simulink model "Sl_H_Infinity_Regulater"  (R2015a)
settings: Solver=FixedStepDiscrete  StartTime=0.0  StopTime=10.0  FixedStep=1  RelTol=1e-3
values from neighbouring files (symbols this model uses):
  kd = c2d(K,0.1)    [Sc_H_Infinity.m]
settings Model: CovSFcnEnable=off  Creator=jordan  LastModifiedBy=Vladislav
settings DataIOCC: SignalLoggingSaveFormat=ModelDataLogs
settings OptimizationCC: ExpressionDepthLimit=2147483647  OptimizeModelRefInitCode=on  LifeSpan=1
settings DebuggingCC: UnderspecifiedInitializationDetection=Classic  MergeDetectMultiDrivingBlocksExec=none  SolverPrmCheckMsg=warning  FcnCallInpInsideContextMsg=UseLocalSettings  StateNameClashWarn=warning
settings RTWCC: SystemTargetFile=ert.tlc  TemplateMakefile=ert_default_tmf  Description=Embedded Coder
settings CodeAppCC: IgnoreCustomStorageClasses=off
settings ERTTargetCC: ParMdlRefBuildCompliant=on  CompOptLevelCompliant=on  ConcurrentExecutionCompliant=on  ERTFirstTimeCompliant=on  SupportContinuousTime=off  SupportVariableSizeSignals=off  ModelStepFunctionPrototypeControlCompliant=on  CPPClassGenCompliant=on  InlinedParameterPlacement=Hierarchical  ERTCustomFileTemplate=example_file_process.tlc

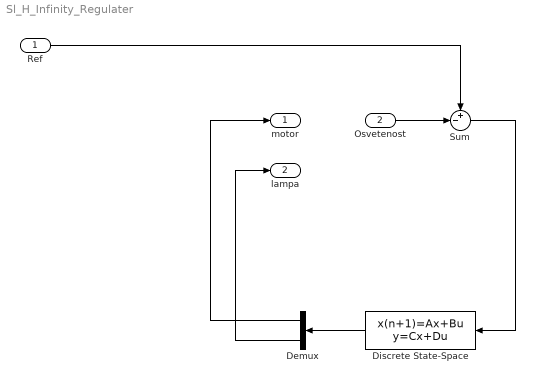
== system Sl_H_Infinity_Regulater ==
  "Ref " : Inport
  "Osvetenost " : Inport  Port=2
  Demux : Demux  Outputs=2
  Discrete State-Space : DiscreteStateSpace  A=kd.a  B=kd.b  C=kd.c  D=kd.d
  Sum : Sum  Inputs=+-|
  motor : Outport
  lampa : Outport  Port=2
  wires:
  Sum/1 -> Discrete State-Space/1
  "Ref "/1 -> Sum/1
  Discrete State-Space/1 -> Demux/1
  Demux/1 -> motor/1
  Demux/2 -> lampa/1
  "Osvetenost "/1 -> Sum/2
